simulink model "VehicleSteering_sim"  (R2019a)
settings: Solver=VariableStepAuto  StartTime=0.0  StopTime=10.0  RelTol=1e-3
InitFcn:
  | Example_VehicleSteering_PP
values from neighbouring files (symbols this model uses):
  A = [0 v0;0 0]    [Example_VehicleSteering_PP.m]
  B = [a*v0/b v0/b]'    [Example_VehicleSteering_PP.m]
  C = eye(2)    [Example_VehicleSteering_PP.m]
  D = [0 0]'    [Example_VehicleSteering_PP.m]
  K = [b*wn^2/v0^2 (2*zeta*wn*b/v0-a*b*wn^2/v0^2)]    [Example_VehicleSteering_PP.m]
  kr = b*wn^2/v0^2    (= 2.77777777778)    [Example_VehicleSteering_PP.m]
settings Model: Creator=jofr  LastModifiedBy=rizwanahmed
settings DataIOCC: ReturnWorkspaceOutputs=off
settings DebuggingCC: ArithmeticOperatorsInVariantConditions=warning
settings SFSimCC: SimUseLocalCustomCode=off
settings RTWCC: RTWUseLocalCustomCode=off

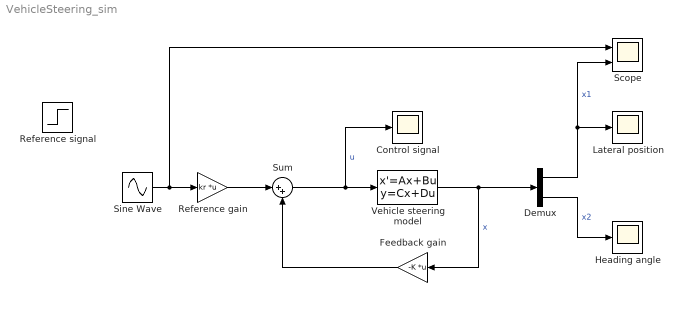
== system VehicleSteering_sim ==
  Control signal : Scope
  Demux : Demux  Outputs=2
  Feedback gain : Gain  Gain=-K  Multiplication=Matrix(K*u)
  Heading angle : Scope
  Lateral position : Scope
  Reference gain : Gain  Gain=kr  Multiplication=Matrix(K*u)
  "Reference signal " : Step  SampleTime=0
  Scope : Scope  NumInputPorts=2
  Sine Wave : Sin  Frequency=2*pi/10  SampleTime=0
  Sum : Sum  Inputs=|++
  Vehicle steering model : StateSpace  A=A  B=B  C=C  D=D  InitialCondition=0
  wires:
  Vehicle steering model/1 -> Demux/1, Feedback gain/1  "x"
  Sum/1 -> Control signal/1, Vehicle steering model/1  "u"
  Feedback gain/1 -> Sum/2
  Reference gain/1 -> Sum/1
  Demux/1 -> Scope/2, Lateral position/1  "x1"
  Demux/2 -> Heading angle/1  "x2"
  Sine Wave/1 -> Scope/1, Reference gain/1
